simulink model "workingGT3nomasknwithcontrol"  (R2024a)
settings: Solver=ode15s  StartTime=0.0  StopTime=3600*48  RelTol=0.0001
model workspace (MAT data in the model file):
  TempGrad = 15
  Ti = 5
  roomarea1 = 20
libraries: fl_lib x2433, nesl_utility x241, SimscapeFluids_lib x137
(part 2 of 41)

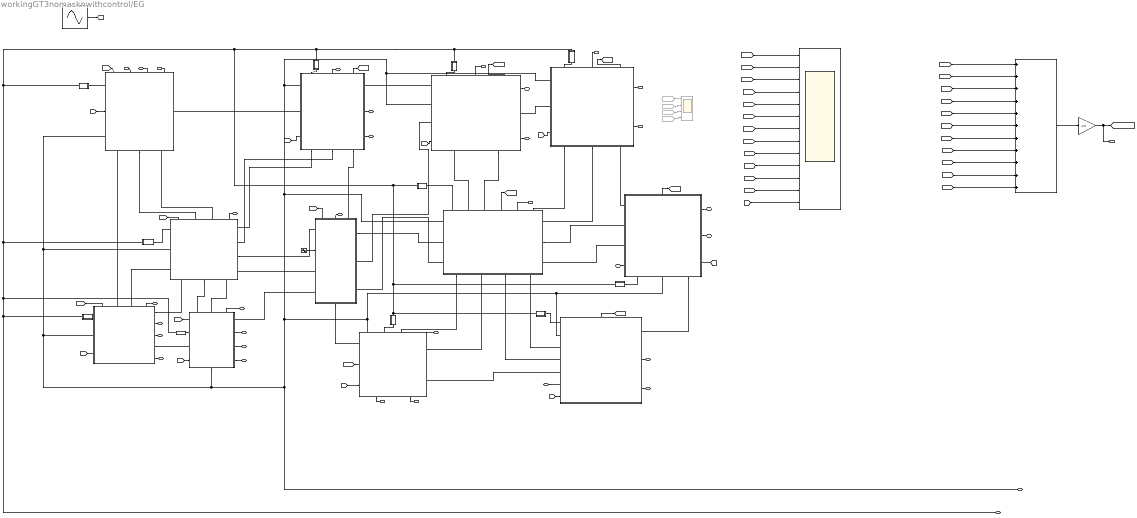
== system workingGT3nomasknwithcontrol/EG ==
  EG : Scope  NumInputPorts=13
  From : From  Commented=on  GotoTag=Troom1
  From1 : From  Commented=on  GotoTag=Troom2
  From2 : From  Commented=on  GotoTag=Troom3
  From3 : From  Commented=on  GotoTag=Troom4
  Pipe to 10 : Subsystem
  Pipe to 11 : Subsystem
  Pipe to 12 : Subsystem
  Pipe to 2 : Subsystem
  Pipe to 4 : Subsystem
  Pipe to 5 : Subsystem
  Pipe to 6 : Subsystem
  Pipe to 7 : Subsystem
  Pipe to 8 : Subsystem
  Pipe to 9a : Subsystem
  Raum1 : Subsystem
      settings: PortSchema="{\"entries\":[{\"content\":{\"sides\":[{\"content\":{\"connectorIds\":[\"LConn1\",\"LConn2\",\"LConn3\"]},\"type\":\"ConnectorPlacement.EquallySpacedRectSide\",\"uuid\":\"258852ae-79b4-4e90-ae22-4154c858ab0a\"},{\"content\":{\"connectorIds\":[\"RConn1\",\"In1\",\"RConn2\",\"RConn3\"],\"side\":\"RIGHT\"},\"type\":\"ConnectorPlacement.EquallySpacedRectSide\",\"uuid\":\"36706832-f330-42ce-9a32-f145cdee4912\"},{\"content\":{\"connectorIds\":[\"LConn4\",\"LConn5\",\"Out1\"],\"side\":\"TOP\"},\"type\":\"ConnectorPlacement.EquallySpacedRectSide\",\"uuid\":\"5cf2347a-3520-447e-9561-2d1c8313f3cf\"},{\"content\":{\"connectorIds\":[\"RConn4\"],\"side\":\"BOTTOM\"},\"type\":\"ConnectorPlacement.EquallySpacedRectSide\",\"uuid\":\"b1588268-8d41-4423-8f6e-2c28bf9b13dc\"}]},\"type\":\"ConnectorPlacement.EquallySpacedConnector\",\"uuid\":\"6bed35e7-1d7a-421b-a1f8-39267ed9017d\"}],\"packageUris\":[\"http://schema.mathworks.com/mf0/Connector/R2020b\"],\"version\":\"1.0\"}"
  Raum10 : Subsystem
      settings: PortSchema="{\"entries\":[{\"content\":{\"sides\":[{\"content\":{\"connectorIds\":[\"LConn1\",\"LConn2\",\"LConn3\",\"In1\"]},\"type\":\"ConnectorPlacement.EquallySpacedRectSide\",\"uuid\":\"258852ae-79b4-4e90-ae22-4154c858ab0a\"},{\"content\":{\"connectorIds\":[\"RConn1\",\"RConn2\",\"RConn3\"],\"side\":\"RIGHT\"},\"type\":\"ConnectorPlacement.EquallySpacedRectSide\",\"uuid\":\"36706832-f330-42ce-9a32-f145cdee4912\"},{\"content\":{\"connectorIds\":[\"LConn4\",\"LConn5\",\"Out1\"],\"side\":\"TOP\"},\"type\":\"ConnectorPlacement.EquallySpacedRectSide\",\"uuid\":\"5cf2347a-3520-447e-9561-2d1c8313f3cf\"},{\"content\":{\"connectorIds\":[\"RConn4\",\"RConn5\"],\"side\":\"BOTTOM\"},\"type\":\"ConnectorPlacement.EquallySpacedRectSide\",\"uuid\":\"b1588268-8d41-4423-8f6e-2c28bf9b13dc\"}]},\"type\":\"ConnectorPlacement.EquallySpacedConnector\",\"uuid\":\"6bed35e7-1d7a-421b-a1f8-39267ed9017d\"}],\"packageUris\":[\"http://schema.mathworks.com/mf0/Connector/R2020b\"],\"version\":\"1.0\"}"
  Raum11 : Subsystem
      settings: PortSchema="{\"entries\":[{\"content\":{\"sides\":[{\"content\":{\"connectorIds\":[\"LConn1\",\"LConn2\",\"In1\"]},\"type\":\"ConnectorPlacement.EquallySpacedRectSide\",\"uuid\":\"258852ae-79b4-4e90-ae22-4154c858ab0a\"},{\"content\":{\"connectorIds\":[\"RConn1\",\"RConn2\",\"RConn3\"],\"side\":\"RIGHT\"},\"type\":\"ConnectorPlacement.EquallySpacedRectSide\",\"uuid\":\"36706832-f330-42ce-9a32-f145cdee4912\"},{\"content\":{\"connectorIds\":[\"LConn3\",\"LConn4\",\"Out1\"],\"side\":\"TOP\"},\"type\":\"ConnectorPlacement.EquallySpacedRectSide\",\"uuid\":\"5cf2347a-3520-447e-9561-2d1c8313f3cf\"},{\"content\":{\"connectorIds\":[\"RConn4\",\"RConn5\",\"RConn6\"],\"side\":\"BOTTOM\"},\"type\":\"ConnectorPlacement.EquallySpacedRectSide\",\"uuid\":\"b1588268-8d41-4423-8f6e-2c28bf9b13dc\"}]},\"type\":\"ConnectorPlacement.EquallySpacedConnector\",\"uuid\":\"6bed35e7-1d7a-421b-a1f8-39267ed9017d\"}],\"packageUris\":[\"http://schema.mathworks.com/mf0/Connector/R2020b\"],\"version\":\"1.0\"}"
  Raum12 : Subsystem
      settings: PortSchema="{\"entries\":[{\"content\":{\"sides\":[{\"content\":{\"connectorIds\":[\"LConn1\",\"In1\",\"LConn2\"]},\"type\":\"ConnectorPlacement.EquallySpacedRectSide\",\"uuid\":\"258852ae-79b4-4e90-ae22-4154c858ab0a\"},{\"content\":{\"connectorIds\":[\"RConn1\"],\"side\":\"RIGHT\"},\"type\":\"ConnectorPlacement.EquallySpacedRectSide\",\"uuid\":\"36706832-f330-42ce-9a32-f145cdee4912\"},{\"content\":{\"connectorIds\":[\"Out1\",\"LConn3\",\"LConn4\",\"LConn5\"],\"side\":\"TOP\"},\"type\":\"ConnectorPlacement.EquallySpacedRectSide\",\"uuid\":\"5cf2347a-3520-447e-9561-2d1c8313f3cf\"},{\"content\":{\"connectorIds\":[\"RConn2\",\"RConn3\",\"RConn4\"],\"side\":\"BOTTOM\"},\"type\":\"ConnectorPlacement.EquallySpacedRectSide\",\"uuid\":\"b1588268-8d41-4423-8f6e-2c28bf9b13dc\"}]},\"type\":\"ConnectorPlacement.EquallySpacedConnector\",\"uuid\":\"6bed35e7-1d7a-421b-a1f8-39267ed9017d\"}],\"packageUris\":[\"http://schema.mathworks.com/mf0/Connector/R2020b\"],\"version\":\"1.0\"}"
  Raum2 : Subsystem
      settings: PortSchema="{\"entries\":[{\"content\":{\"sides\":[{\"content\":{\"connectorIds\":[\"LConn1\",\"LConn2\",\"LConn3\"]},\"type\":\"ConnectorPlacement.EquallySpacedRectSide\",\"uuid\":\"258852ae-79b4-4e90-ae22-4154c858ab0a\"},{\"content\":{\"connectorIds\":[\"RConn1\",\"RConn2\",\"RConn3\",\"RConn4\"],\"side\":\"RIGHT\"},\"type\":\"ConnectorPlacement.EquallySpacedRectSide\",\"uuid\":\"36706832-f330-42ce-9a32-f145cdee4912\"},{\"content\":{\"connectorIds\":[\"Out1\",\"LConn4\",\"LConn5\",\"LConn6\"],\"side\":\"TOP\"},\"type\":\"ConnectorPlacement.EquallySpacedRectSide\",\"uuid\":\"5cf2347a-3520-447e-9561-2d1c8313f3cf\"},{\"content\":{\"connectorIds\":[\"RConn5\",\"RConn6\",\"RConn7\"],\"side\":\"BOTTOM\"},\"type\":\"ConnectorPlacement.EquallySpacedRectSide\",\"uuid\":\"b1588268-8d41-4423-8f6e-2c28bf9b13dc\"}]},\"type\":\"ConnectorPlacement.EquallySpacedConnector\",\"uuid\":\"6bed35e7-1d7a-421b-a1f8-39267ed9017d\"}],\"packageUris\":[\"http://schema.mathworks.com/mf0/Connector/R2020b\"],\"version\":\"1.0\"}"
  Raum3 : Subsystem
      settings: PortSchema="{\"entries\":[{\"content\":{\"sides\":[{\"content\":{\"connectorIds\":[\"LConn1\",\"LConn2\",\"In1\"]},\"type\":\"ConnectorPlacement.EquallySpacedRectSide\",\"uuid\":\"258852ae-79b4-4e90-ae22-4154c858ab0a\"},{\"content\":{\"connectorIds\":[\"RConn1\",\"RConn2\",\"RConn3\",\"RConn4\",\"RConn5\"],\"side\":\"RIGHT\"},\"type\":\"ConnectorPlacement.EquallySpacedRectSide\",\"uuid\":\"36706832-f330-42ce-9a32-f145cdee4912\"},{\"content\":{\"connectorIds\":[\"Out1\",\"LConn3\",\"LConn4\",\"LConn5\"],\"side\":\"TOP\"},\"type\":\"ConnectorPlacement.EquallySpacedRectSide\",\"uuid\":\"5cf2347a-3520-447e-9561-2d1c8313f3cf\"},{\"content\":{\"side\":\"BOTTOM\"},\"type\":\"ConnectorPlacement.EquallySpacedRectSide\",\"uuid\":\"b1588268-8d41-4423-8f6e-2c28bf9b13dc\"}]},\"type\":\"ConnectorPlacement.EquallySpacedConnector\",\"uuid\":\"6bed35e7-1d7a-421b-a1f8-39267ed9017d\"}],\"packageUris\":[\"http://schema.mathworks.com/mf0/Connector/R2020b\"],\"version\":\"1.0\"}"
  Raum4 : Subsystem
      settings: PortSchema="{\"entries\":[{\"content\":{\"sides\":[{\"content\":{\"connectorIds\":[\"Out1\",\"LConn1\",\"LConn2\",\"In1\"]},\"type\":\"ConnectorPlacement.EquallySpacedRectSide\",\"uuid\":\"258852ae-79b4-4e90-ae22-4154c858ab0a\"},{\"content\":{\"connectorIds\":[\"RConn1\",\"RConn2\",\"RConn3\",\"RConn4\"],\"side\":\"RIGHT\"},\"type\":\"ConnectorPlacement.EquallySpacedRectSide\",\"uuid\":\"36706832-f330-42ce-9a32-f145cdee4912\"},{\"content\":{\"connectorIds\":[\"LConn3\",\"LConn4\",\"LConn5\"],\"side\":\"TOP\"},\"type\":\"ConnectorPlacement.EquallySpacedRectSide\",\"uuid\":\"5cf2347a-3520-447e-9561-2d1c8313f3cf\"},{\"content\":{\"connectorIds\":[\"RConn5\"],\"side\":\"BOTTOM\"},\"type\":\"ConnectorPlacement.EquallySpacedRectSide\",\"uuid\":\"b1588268-8d41-4423-8f6e-2c28bf9b13dc\"}]},\"type\":\"ConnectorPlacement.EquallySpacedConnector\",\"uuid\":\"6bed35e7-1d7a-421b-a1f8-39267ed9017d\"}],\"packageUris\":[\"http://schema.mathworks.com/mf0/Connector/R2020b\"],\"version\":\"1.0\"}"
  Raum5 : Subsystem
      settings: PortSchema="{\"entries\":[{\"content\":{\"sides\":[{\"content\":{\"connectorIds\":[\"LConn1\",\"LConn2\",\"LConn3\",\"LConn4\"]},\"type\":\"ConnectorPlacement.EquallySpacedRectSide\",\"uuid\":\"258852ae-79b4-4e90-ae22-4154c858ab0a\"},{\"content\":{\"connectorIds\":[\"RConn1\",\"RConn2\",\"In1\"],\"side\":\"RIGHT\"},\"type\":\"ConnectorPlacement.EquallySpacedRectSide\",\"uuid\":\"36706832-f330-42ce-9a32-f145cdee4912\"},{\"content\":{\"connectorIds\":[\"Out1\"],\"side\":\"TOP\"},\"type\":\"ConnectorPlacement.EquallySpacedRectSide\",\"uuid\":\"5cf2347a-3520-447e-9561-2d1c8313f3cf\"},{\"content\":{\"connectorIds\":[\"RConn3\",\"RConn4\",\"RConn5\"],\"side\":\"BOTTOM\"},\"type\":\"ConnectorPlacement.EquallySpacedRectSide\",\"uuid\":\"b1588268-8d41-4423-8f6e-2c28bf9b13dc\"}]},\"type\":\"ConnectorPlacement.EquallySpacedConnector\",\"uuid\":\"6bed35e7-1d7a-421b-a1f8-39267ed9017d\"}],\"packageUris\":[\"http://schema.mathworks.com/mf0/Connector/R2020b\"],\"version\":\"1.0\"}"
  Raum6 : Subsystem
      settings: PortSchema="{\"entries\":[{\"content\":{\"sides\":[{\"content\":{\"connectorIds\":[\"LConn1\",\"LConn2\",\"LConn3\",\"LConn4\",\"LConn5\",\"LConn6\",\"In1\"]},\"type\":\"ConnectorPlacement.EquallySpacedRectSide\",\"uuid\":\"258852ae-79b4-4e90-ae22-4154c858ab0a\"},{\"content\":{\"connectorIds\":[\"RConn1\",\"RConn2\",\"RConn3\"],\"side\":\"RIGHT\"},\"type\":\"ConnectorPlacement.EquallySpacedRectSide\",\"uuid\":\"36706832-f330-42ce-9a32-f145cdee4912\"},{\"content\":{\"connectorIds\":[\"Out1\"],\"side\":\"TOP\"},\"type\":\"ConnectorPlacement.EquallySpacedRectSide\",\"uuid\":\"5cf2347a-3520-447e-9561-2d1c8313f3cf\"},{\"content\":{\"side\":\"BOTTOM\"},\"type\":\"ConnectorPlacement.EquallySpacedRectSide\",\"uuid\":\"b1588268-8d41-4423-8f6e-2c28bf9b13dc\"}]},\"type\":\"ConnectorPlacement.EquallySpacedConnector\",\"uuid\":\"6bed35e7-1d7a-421b-a1f8-39267ed9017d\"}],\"packageUris\":[\"http://schema.mathworks.com/mf0/Connector/R2020b\"],\"version\":\"1.0\"}"
  Raum7 : Subsystem
      settings: PortSchema="{\"entries\":[{\"content\":{\"sides\":[{\"content\":{\"connectorIds\":[\"LConn1\",\"LConn2\",\"LConn3\"]},\"type\":\"ConnectorPlacement.EquallySpacedRectSide\",\"uuid\":\"258852ae-79b4-4e90-ae22-4154c858ab0a\"},{\"content\":{\"connectorIds\":[\"RConn1\",\"RConn2\",\"RConn3\"],\"side\":\"RIGHT\"},\"type\":\"ConnectorPlacement.EquallySpacedRectSide\",\"uuid\":\"36706832-f330-42ce-9a32-f145cdee4912\"},{\"content\":{\"connectorIds\":[\"LConn4\",\"LConn5\",\"LConn6\",\"Out1\",\"LConn7\",\"LConn8\"],\"side\":\"TOP\"},\"type\":\"ConnectorPlacement.EquallySpacedRectSide\",\"uuid\":\"5cf2347a-3520-447e-9561-2d1c8313f3cf\"},{\"content\":{\"connectorIds\":[\"RConn4\",\"RConn5\",\"RConn6\",\"RConn7\"],\"side\":\"BOTTOM\"},\"type\":\"ConnectorPlacement.EquallySpacedRectSide\",\"uuid\":\"b1588268-8d41-4423-8f6e-2c28bf9b13dc\"}]},\"type\":\"ConnectorPlacement.EquallySpacedConnector\",\"uuid\":\"6bed35e7-1d7a-421b-a1f8-39267ed9017d\"}],\"packageUris\":[\"http://schema.mathworks.com/mf0/Connector/R2020b\"],\"version\":\"1.0\"}"
  Raum8 : Subsystem
      settings: PortSchema="{\"entries\":[{\"content\":{\"sides\":[{\"content\":{\"connectorIds\":[\"LConn1\",\"Out1\",\"In1\"]},\"type\":\"ConnectorPlacement.EquallySpacedRectSide\",\"uuid\":\"258852ae-79b4-4e90-ae22-4154c858ab0a\"},{\"content\":{\"connectorIds\":[\"RConn1\",\"RConn2\"],\"side\":\"RIGHT\"},\"type\":\"ConnectorPlacement.EquallySpacedRectSide\",\"uuid\":\"36706832-f330-42ce-9a32-f145cdee4912\"},{\"content\":{\"connectorIds\":[\"LConn2\",\"LConn3\",\"LConn4\",\"LConn5\"],\"side\":\"TOP\"},\"type\":\"ConnectorPlacement.EquallySpacedRectSide\",\"uuid\":\"5cf2347a-3520-447e-9561-2d1c8313f3cf\"},{\"content\":{\"connectorIds\":[\"RConn3\",\"RConn4\"],\"side\":\"BOTTOM\"},\"type\":\"ConnectorPlacement.EquallySpacedRectSide\",\"uuid\":\"b1588268-8d41-4423-8f6e-2c28bf9b13dc\"}]},\"type\":\"ConnectorPlacement.EquallySpacedConnector\",\"uuid\":\"6bed35e7-1d7a-421b-a1f8-39267ed9017d\"}],\"packageUris\":[\"http://schema.mathworks.com/mf0/Connector/R2020b\"],\"version\":\"1.0\"}"
  Raum9 : Subsystem
      settings: PortSchema="{\"entries\":[{\"content\":{\"sides\":[{\"content\":{\"connectorIds\":[\"LConn1\",\"LConn2\",\"In1\"]},\"type\":\"ConnectorPlacement.EquallySpacedRectSide\",\"uuid\":\"258852ae-79b4-4e90-ae22-4154c858ab0a\"},{\"content\":{\"connectorIds\":[\"RConn1\",\"RConn2\"],\"side\":\"RIGHT\"},\"type\":\"ConnectorPlacement.EquallySpacedRectSide\",\"uuid\":\"36706832-f330-42ce-9a32-f145cdee4912\"},{\"content\":{\"connectorIds\":[\"LConn3\",\"LConn4\",\"Out1\"],\"side\":\"TOP\"},\"type\":\"ConnectorPlacement.EquallySpacedRectSide\",\"uuid\":\"5cf2347a-3520-447e-9561-2d1c8313f3cf\"},{\"content\":{\"connectorIds\":[\"RConn3\",\"RConn4\",\"RConn5\"],\"side\":\"BOTTOM\"},\"type\":\"ConnectorPlacement.EquallySpacedRectSide\",\"uuid\":\"b1588268-8d41-4423-8f6e-2c28bf9b13dc\"}]},\"type\":\"ConnectorPlacement.EquallySpacedConnector\",\"uuid\":\"6bed35e7-1d7a-421b-a1f8-39267ed9017d\"}],\"packageUris\":[\"http://schema.mathworks.com/mf0/Connector/R2020b\"],\"version\":\"1.0\"}"
  RaumTemperaturverlauf : Scope  Commented=on  NumInputPorts=4
  Sum of Elements : Sum  Inputs=+++++++++++
  Tatm11 : Sin  Amplitude=12  Frequency=2*pi/(24*3600)  Phase=-0.5*pi  SampleTime=0
  Tatm12 : Sin  Amplitude=7  Bias=5  Frequency=2*pi/(24*3600)  SampleTime=0
  TavgEG : Gain  Gain=1/11
  pipe to 3 : Subsystem
  hot water in : PMIOPort  Side=Left
  Y-1 : PMIOPort  Port=2  Side=Right
  Y-3 : PMIOPort  Port=3  Side=Right
  Y-4 : PMIOPort  Port=4  Side=Right
  Y-5 : PMIOPort  Port=5  Side=Right
  Y-6 : PMIOPort  Port=6  Side=Right
  Y-8 : PMIOPort  Port=7  Side=Right
  Y-7 : PMIOPort  Port=8  Side=Right
  Y-9 : PMIOPort  Port=9  Side=Right
  Y-10 : PMIOPort  Port=10  Side=Right
  Y-11 : PMIOPort  Port=11  Side=Right
  Y-12 : PMIOPort  Port=12  Side=Right
  Y-13 : PMIOPort  Port=13  Side=Right
  Y-14 : PMIOPort  Port=14  Side=Right
  Y-15 : PMIOPort  Port=15  Side=Right
  Y-16 : PMIOPort  Port=16  Side=Right
  Y-17 : PMIOPort  Port=17  Side=Right
  Y-18 : PMIOPort  Port=18  Side=Right
  Y-19 : PMIOPort  Port=19  Side=Right
  Y-20 : PMIOPort  Port=20  Side=Right
  Y-21 : PMIOPort  Port=21  Side=Right
  Hot Water Out1 : PMIOPort  Port=22  Side=Right
  Y-6 Flur12OG2 : PMIOPort  Port=23  Side=Right
  Y-Flur11OG2 : PMIOPort  Port=24  Side=Right
  Y-Flur10OG2 : PMIOPort  Port=25  Side=Right
  Y-Flur9OG2 : PMIOPort  Port=26  Side=Right
  Y-Flur8OG2 : PMIOPort  Port=27  Side=Right
  Y-Flur7OG2 : PMIOPort  Port=28  Side=Right
  Y-Flur6OG2 : PMIOPort  Port=29  Side=Right
  Y-Flur5OG2 : PMIOPort  Port=30  Side=Right
  Y-Flur4OG2 : PMIOPort  Port=31  Side=Right
  Y-Flur3OG2 : PMIOPort  Port=32  Side=Right
  Y-Flur2OG2 : PMIOPort  Port=33  Side=Right
  Y-Flur1OG2 : PMIOPort  Port=34  Side=Right
  Output : Outport
  wires:
  Raum9/1(Troom) -> [Traum9]
  [Traum4] -> EG/4
  [Traum10] -> EG/10
  [Tatm] -> Raum11/1(Tatm)
  Raum6/1(Troom) -> [Traum6]
  [Traum5] -> EG/5
  [Traum7] -> EG/7
  [Tatm] -> Raum9/1(Tatm)
  Raum7/1(Troom) -> [Traum7]
  [Traum9] -> EG/9
  From/1 -> RaumTemperaturverlauf/1
  [Traum12] -> EG/12
  Raum11/1(Troom) -> [Troom11]
  [Traum6] -> EG/6
  From2/1 -> RaumTemperaturverlauf/3
  Raum2/1(Troom) -> [Traum2]
  From3/1 -> RaumTemperaturverlauf/4
  [Tatm] -> Raum10/1(Tatm)
  Tatm11/1 -> Raum1/1(Tatm)
  [Tatm] -> Raum5/1(Tatm)
  [Tatm] -> Raum3/1(Tatm)
  [Traum1] -> EG/1
  [Tatm] -> Raum4/1(Tatm)
  From1/1 -> RaumTemperaturverlauf/2
  [Traum2] -> EG/2
  Raum3/1(Troom) -> [Traum3]
  Raum10/1(Troom) -> [Traum10]
  Raum1/1(Troom) -> [Traum1]
  [Tatm] -> Raum6/1(Tatm)
  [Traum3] -> EG/3
  [Tatm] -> Raum8/1(Tatm)
  Raum4/1(Troom) -> [Traum4]
  Raum5/1(Troom) -> [Traum5]
  [Traum8] -> EG/8
  [Troom11] -> EG/11
  Raum8/1(Troom) -> [Traum8]
  Raum12/1(Troom) -> [Traum12]
  [Tatm] -> Raum12/1(Tatm)
  Tatm12/1 -> [Tatm]
  [Troom11] -> Sum of Elements/10
  [Traum8] -> Sum of Elements/7
  [Traum3] -> Sum of Elements/2
  [Traum2] -> Sum of Elements/1
  [Traum6] -> Sum of Elements/5
  [Traum12] -> Sum of Elements/11
  [Traum9] -> Sum of Elements/8
  [Traum7] -> Sum of Elements/6
  [Traum5] -> Sum of Elements/4
  [Traum10] -> Sum of Elements/9
  [Traum4] -> Sum of Elements/3
  Sum of Elements/1 -> TavgEG/1
  TavgEG/1 -> Output/1, [TavgEG]
  [TavgEG] -> EG/13
  connections:
  Raum6/LConn5 -- Raum8/RConn2
  Raum3/LConn2 -- Raum2/LConn2 -- Raum12/LConn2 -- Raum5/RConn4 -- Raum6/LConn2 -- Raum8/LConn2 -- Raum11/LConn1 -- Raum9/LConn1 -- Raum10/LConn2 -- Raum7/LConn1 -- Hot Water Out1/RConn1 -- Raum4/RConn5
  Raum5/RConn5 -- Raum6/RConn1
  Raum7/RConn6 -- Raum6/LConn4
  Pipe to 6/RConn1 -- Raum6/LConn1
  Raum11/RConn2 -- Y-3/RConn1
  Raum1/RConn2 -- Raum2/RConn4
  Pipe to 12/RConn1 -- Raum12/LConn1
  Pipe to 7/RConn1 -- Raum7/LConn4
  Raum11/LConn2 -- Raum12/RConn1
  Pipe to 4/LConn1 -- Pipe to 2/LConn1 -- Pipe to 11/LConn1 -- Pipe to 10/LConn1 -- Pipe to 9a/LConn1 -- Pipe to 7/LConn1 -- Pipe to 6/LConn1 -- Pipe to 8/LConn1 -- Pipe to 5/LConn1 -- Pipe to 12/LConn1 -- hot water in/RConn1 -- pipe to 3/LConn1
  Raum3/LConn4 -- Raum2/LConn3
  Raum4/LConn4 -- Raum2/RConn7
  Raum10/RConn3 -- Y-9/RConn1
  Raum11/RConn6 -- Raum1/LConn4
  Raum9/LConn3 -- Pipe to 9a/RConn1
  Raum5/LConn1 -- Raum9/RConn5
  Pipe to 4/RConn1 -- Raum4/LConn1
  Raum6/RConn2 -- Y-16/RConn1
  Raum4/RConn4 -- Y-17/RConn1
  Raum3/RConn5 -- Y-18/RConn1
  Raum7/RConn7 -- Raum6/LConn3
  Pipe to 8/RConn1 -- Raum8/LConn3
  Pipe to 11/RConn1 -- Raum11/LConn3
  Raum9/RConn4 -- Raum7/RConn1
  Raum10/LConn1 -- Raum11/RConn1
  Raum8/RConn3 -- Y-20/RConn1
  Raum2/LConn5 -- Raum12/RConn4
  Raum7/LConn3 -- Raum1/LConn3
  Pipe to 10/RConn1 -- Raum10/LConn4
  Raum10/RConn1 -- Y-1/RConn1
  Raum12/LConn5 -- Y-7/RConn1
  pipe to 3/RConn1 -- Raum3/LConn1
  Raum11/RConn3 -- Y-8/RConn1
  Raum1/RConn4 -- Raum8/LConn1
  Raum9/LConn2 -- Raum10/RConn2
  Raum5/LConn3 -- Raum7/RConn3
  Raum9/RConn1 -- Y-6/RConn1
  Raum2/RConn6 -- Raum4/LConn3
  Raum7/RConn4 -- Raum8/LConn4
  Raum3/LConn3 -- Raum12/RConn2
  Raum10/LConn3 -- Raum1/LConn2
  Pipe to 2/RConn1 -- Raum2/LConn1
  Raum12/RConn3 -- Raum2/LConn4
  Raum10/RConn5 -- Raum7/LConn6
  Raum7/RConn2 -- Raum5/LConn2
  Raum11/RConn4 -- Raum2/RConn1
  Raum3/RConn1 -- Raum2/RConn5
  Raum9/RConn3 -- Raum7/LConn8
  Raum3/RConn4 -- Raum4/LConn2
  Pipe to 5/RConn1 -- Raum5/RConn3
  Raum1/RConn3 -- Raum4/RConn1
  Raum1/LConn1 -- Raum7/LConn2
  Raum11/RConn5 -- Raum2/RConn2
  Raum8/RConn1 -- Raum7/RConn5
  Raum7/LConn5 -- Raum10/RConn4
  Raum2/RConn3 -- Raum1/RConn1
  Raum4/RConn3 -- Y-15/RConn1
  Raum5/RConn1 -- Y-10/RConn1
  Raum9/RConn2 -- Y-4/RConn1
  Raum5/RConn2 -- Y-11/RConn1
  Raum8/RConn4 -- Y-21/RConn1
  Raum12/LConn3 -- Y-5/RConn1
  Raum12/LConn4 -- Y-6 Flur12OG2/RConn1
  Raum3/RConn3 -- Y-14/RConn1
  Raum3/RConn2 -- Y-12/RConn1
  Raum4/RConn2 -- Y-13/RConn1
  Raum6/RConn3 -- Y-19/RConn1
  Raum11/LConn4 -- Y-Flur11OG2/RConn1
  Raum10/LConn5 -- Y-Flur10OG2/RConn1
  Raum9/LConn4 -- Y-Flur9OG2/RConn1
  Y-Flur5OG2/RConn1 -- Raum5/LConn4
  Raum7/LConn7 -- Y-Flur7OG2/RConn1
  Y-Flur6OG2/RConn1 -- Raum6/LConn6
  Y-Flur8OG2/RConn1 -- Raum8/LConn5
  Raum1/LConn5 -- Y-Flur1OG2/RConn1
  Y-Flur4OG2/RConn1 -- Raum4/LConn5
  Raum3/LConn5 -- Y-Flur3OG2/RConn1
  Raum2/LConn6 -- Y-Flur2OG2/RConn1

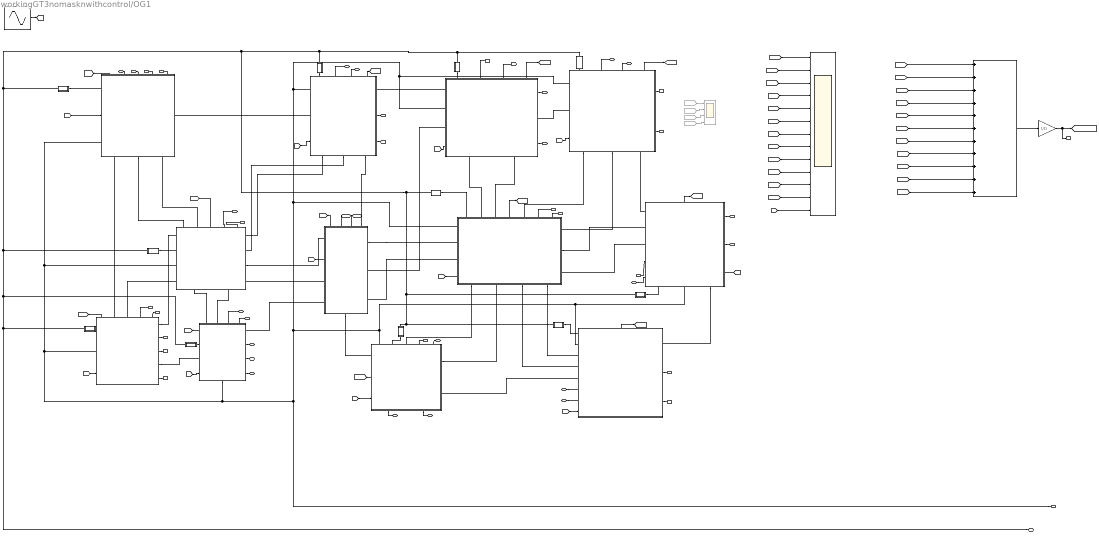
== system workingGT3nomasknwithcontrol/OG1 ==
  From : From  Commented=on  GotoTag=Troom1
  From1 : From  Commented=on  GotoTag=Troom2
  From2 : From  Commented=on  GotoTag=Troom3
  From3 : From  Commented=on  GotoTag=Troom4
  OG1 : Scope  NumInputPorts=13
  Pipe to 10 : Subsystem
  Pipe to 11 : Subsystem
  Pipe to 12 : Subsystem
  Pipe to 2 : Subsystem
  Pipe to 4 : Subsystem
  Pipe to 5 : Subsystem
  Pipe to 6 : Subsystem
  Pipe to 7 : Subsystem
  Pipe to 8 : Subsystem
  Pipe to 9a : Subsystem
  Raum1 : Subsystem
      settings: PortSchema="{\"entries\":[{\"content\":{\"sides\":[{\"content\":{\"connectorIds\":[\"LConn1\",\"LConn2\",\"LConn3\"]},\"type\":\"ConnectorPlacement.EquallySpacedRectSide\",\"uuid\":\"258852ae-79b4-4e90-ae22-4154c858ab0a\"},{\"content\":{\"connectorIds\":[\"RConn1\",\"In1\",\"RConn2\",\"RConn3\"],\"side\":\"RIGHT\"},\"type\":\"ConnectorPlacement.EquallySpacedRectSide\",\"uuid\":\"36706832-f330-42ce-9a32-f145cdee4912\"},{\"content\":{\"connectorIds\":[\"LConn4\",\"LConn5\",\"LConn6\",\"Out1\"],\"side\":\"TOP\"},\"type\":\"ConnectorPlacement.EquallySpacedRectSide\",\"uuid\":\"5cf2347a-3520-447e-9561-2d1c8313f3cf\"},{\"content\":{\"connectorIds\":[\"RConn4\"],\"side\":\"BOTTOM\"},\"type\":\"ConnectorPlacement.EquallySpacedRectSide\",\"uuid\":\"b1588268-8d41-4423-8f6e-2c28bf9b13dc\"}]},\"type\":\"ConnectorPlacement.EquallySpacedConnector\",\"uuid\":\"6bed35e7-1d7a-421b-a1f8-39267ed9017d\"}],\"packageUris\":[\"http://schema.mathworks.com/mf0/Connector/R2020b\"],\"version\":\"1.0\"}"
  Raum10 : Subsystem
      settings: PortSchema="{\"entries\":[{\"content\":{\"sides\":[{\"content\":{\"connectorIds\":[\"LConn1\",\"LConn2\",\"LConn3\",\"In1\"]},\"type\":\"ConnectorPlacement.EquallySpacedRectSide\",\"uuid\":\"258852ae-79b4-4e90-ae22-4154c858ab0a\"},{\"content\":{\"connectorIds\":[\"RConn1\",\"RConn2\",\"RConn3\"],\"side\":\"RIGHT\"},\"type\":\"ConnectorPlacement.EquallySpacedRectSide\",\"uuid\":\"36706832-f330-42ce-9a32-f145cdee4912\"},{\"content\":{\"connectorIds\":[\"LConn4\",\"LConn5\",\"LConn6\",\"Out1\"],\"side\":\"TOP\"},\"type\":\"ConnectorPlacement.EquallySpacedRectSide\",\"uuid\":\"5cf2347a-3520-447e-9561-2d1c8313f3cf\"},{\"content\":{\"connectorIds\":[\"RConn4\",\"RConn5\"],\"side\":\"BOTTOM\"},\"type\":\"ConnectorPlacement.EquallySpacedRectSide\",\"uuid\":\"b1588268-8d41-4423-8f6e-2c28bf9b13dc\"}]},\"type\":\"ConnectorPlacement.EquallySpacedConnector\",\"uuid\":\"6bed35e7-1d7a-421b-a1f8-39267ed9017d\"}],\"packageUris\":[\"http://schema.mathworks.com/mf0/Connector/R2020b\"],\"version\":\"1.0\"}"
  Raum11 : Subsystem
      settings: PortSchema="{\"entries\":[{\"content\":{\"sides\":[{\"content\":{\"connectorIds\":[\"LConn1\",\"LConn2\",\"In1\"]},\"type\":\"ConnectorPlacement.EquallySpacedRectSide\",\"uuid\":\"258852ae-79b4-4e90-ae22-4154c858ab0a\"},{\"content\":{\"connectorIds\":[\"RConn1\",\"RConn2\",\"RConn3\"],\"side\":\"RIGHT\"},\"type\":\"ConnectorPlacement.EquallySpacedRectSide\",\"uuid\":\"36706832-f330-42ce-9a32-f145cdee4912\"},{\"content\":{\"connectorIds\":[\"LConn3\",\"LConn4\",\"LConn5\",\"Out1\"],\"side\":\"TOP\"},\"type\":\"ConnectorPlacement.EquallySpacedRectSide\",\"uuid\":\"5cf2347a-3520-447e-9561-2d1c8313f3cf\"},{\"content\":{\"connectorIds\":[\"RConn4\",\"RConn5\",\"RConn6\"],\"side\":\"BOTTOM\"},\"type\":\"ConnectorPlacement.EquallySpacedRectSide\",\"uuid\":\"b1588268-8d41-4423-8f6e-2c28bf9b13dc\"}]},\"type\":\"ConnectorPlacement.EquallySpacedConnector\",\"uuid\":\"6bed35e7-1d7a-421b-a1f8-39267ed9017d\"}],\"packageUris\":[\"http://schema.mathworks.com/mf0/Connector/R2020b\"],\"version\":\"1.0\"}"
  Raum12 : Subsystem
      settings: PortSchema="{\"entries\":[{\"content\":{\"sides\":[{\"content\":{\"connectorIds\":[\"LConn1\",\"In1\",\"LConn2\"]},\"type\":\"ConnectorPlacement.EquallySpacedRectSide\",\"uuid\":\"258852ae-79b4-4e90-ae22-4154c858ab0a\"},{\"content\":{\"connectorIds\":[\"RConn1\"],\"side\":\"RIGHT\"},\"type\":\"ConnectorPlacement.EquallySpacedRectSide\",\"uuid\":\"36706832-f330-42ce-9a32-f145cdee4912\"},{\"content\":{\"connectorIds\":[\"Out1\",\"LConn3\",\"LConn4\",\"LConn5\",\"LConn6\"],\"side\":\"TOP\"},\"type\":\"ConnectorPlacement.EquallySpacedRectSide\",\"uuid\":\"5cf2347a-3520-447e-9561-2d1c8313f3cf\"},{\"content\":{\"connectorIds\":[\"RConn2\",\"RConn3\",\"RConn4\"],\"side\":\"BOTTOM\"},\"type\":\"ConnectorPlacement.EquallySpacedRectSide\",\"uuid\":\"b1588268-8d41-4423-8f6e-2c28bf9b13dc\"}]},\"type\":\"ConnectorPlacement.EquallySpacedConnector\",\"uuid\":\"6bed35e7-1d7a-421b-a1f8-39267ed9017d\"}],\"packageUris\":[\"http://schema.mathworks.com/mf0/Connector/R2020b\"],\"version\":\"1.0\"}"
  Raum2 : Subsystem
      settings: PortSchema="{\"entries\":[{\"content\":{\"sides\":[{\"content\":{\"connectorIds\":[\"LConn1\",\"LConn2\",\"LConn3\",\"LConn4\"]},\"type\":\"ConnectorPlacement.EquallySpacedRectSide\",\"uuid\":\"258852ae-79b4-4e90-ae22-4154c858ab0a\"},{\"content\":{\"connectorIds\":[\"RConn1\",\"RConn2\",\"RConn3\",\"RConn4\"],\"side\":\"RIGHT\"},\"type\":\"ConnectorPlacement.EquallySpacedRectSide\",\"uuid\":\"36706832-f330-42ce-9a32-f145cdee4912\"},{\"content\":{\"connectorIds\":[\"LConn5\",\"LConn6\",\"Out1\",\"LConn7\",\"LConn8\"],\"side\":\"TOP\"},\"type\":\"ConnectorPlacement.EquallySpacedRectSide\",\"uuid\":\"5cf2347a-3520-447e-9561-2d1c8313f3cf\"},{\"content\":{\"connectorIds\":[\"RConn5\",\"RConn6\"],\"side\":\"BOTTOM\"},\"type\":\"ConnectorPlacement.EquallySpacedRectSide\",\"uuid\":\"b1588268-8d41-4423-8f6e-2c28bf9b13dc\"}]},\"type\":\"ConnectorPlacement.EquallySpacedConnector\",\"uuid\":\"6bed35e7-1d7a-421b-a1f8-39267ed9017d\"}],\"packageUris\":[\"http://schema.mathworks.com/mf0/Connector/R2020b\"],\"version\":\"1.0\"}"
  Raum3 : Subsystem
      settings: PortSchema="{\"entries\":[{\"content\":{\"sides\":[{\"content\":{\"connectorIds\":[\"LConn1\",\"LConn2\",\"In1\"]},\"type\":\"ConnectorPlacement.EquallySpacedRectSide\",\"uuid\":\"258852ae-79b4-4e90-ae22-4154c858ab0a\"},{\"content\":{\"connectorIds\":[\"RConn1\",\"RConn2\",\"RConn3\",\"RConn4\",\"RConn5\"],\"side\":\"RIGHT\"},\"type\":\"ConnectorPlacement.EquallySpacedRectSide\",\"uuid\":\"36706832-f330-42ce-9a32-f145cdee4912\"},{\"content\":{\"connectorIds\":[\"Out1\",\"LConn3\",\"LConn4\",\"LConn5\",\"LConn6\"],\"side\":\"TOP\"},\"type\":\"ConnectorPlacement.EquallySpacedRectSide\",\"uuid\":\"5cf2347a-3520-447e-9561-2d1c8313f3cf\"},{\"content\":{\"side\":\"BOTTOM\"},\"type\":\"ConnectorPlacement.EquallySpacedRectSide\",\"uuid\":\"b1588268-8d41-4423-8f6e-2c28bf9b13dc\"}]},\"type\":\"ConnectorPlacement.EquallySpacedConnector\",\"uuid\":\"6bed35e7-1d7a-421b-a1f8-39267ed9017d\"}],\"packageUris\":[\"http://schema.mathworks.com/mf0/Connector/R2020b\"],\"version\":\"1.0\"}"
  Raum4 : Subsystem
      settings: PortSchema="{\"entries\":[{\"content\":{\"sides\":[{\"content\":{\"connectorIds\":[\"Out1\",\"LConn1\",\"LConn2\",\"In1\"]},\"type\":\"ConnectorPlacement.EquallySpacedRectSide\",\"uuid\":\"258852ae-79b4-4e90-ae22-4154c858ab0a\"},{\"content\":{\"connectorIds\":[\"RConn1\",\"RConn2\",\"RConn3\",\"RConn4\"],\"side\":\"RIGHT\"},\"type\":\"ConnectorPlacement.EquallySpacedRectSide\",\"uuid\":\"36706832-f330-42ce-9a32-f145cdee4912\"},{\"content\":{\"connectorIds\":[\"LConn3\",\"LConn4\",\"LConn5\",\"LConn6\"],\"side\":\"TOP\"},\"type\":\"ConnectorPlacement.EquallySpacedRectSide\",\"uuid\":\"5cf2347a-3520-447e-9561-2d1c8313f3cf\"},{\"content\":{\"connectorIds\":[\"RConn5\"],\"side\":\"BOTTOM\"},\"type\":\"ConnectorPlacement.EquallySpacedRectSide\",\"uuid\":\"b1588268-8d41-4423-8f6e-2c28bf9b13dc\"}]},\"type\":\"ConnectorPlacement.EquallySpacedConnector\",\"uuid\":\"6bed35e7-1d7a-421b-a1f8-39267ed9017d\"}],\"packageUris\":[\"http://schema.mathworks.com/mf0/Connector/R2020b\"],\"version\":\"1.0\"}"
  Raum5 : Subsystem
      settings: PortSchema="{\"entries\":[{\"content\":{\"sides\":[{\"content\":{\"connectorIds\":[\"LConn1\",\"LConn2\",\"LConn3\",\"LConn4\",\"LConn5\"]},\"type\":\"ConnectorPlacement.EquallySpacedRectSide\",\"uuid\":\"258852ae-79b4-4e90-ae22-4154c858ab0a\"},{\"content\":{\"connectorIds\":[\"RConn1\",\"RConn2\",\"In1\"],\"side\":\"RIGHT\"},\"type\":\"ConnectorPlacement.EquallySpacedRectSide\",\"uuid\":\"36706832-f330-42ce-9a32-f145cdee4912\"},{\"content\":{\"connectorIds\":[\"Out1\"],\"side\":\"TOP\"},\"type\":\"ConnectorPlacement.EquallySpacedRectSide\",\"uuid\":\"5cf2347a-3520-447e-9561-2d1c8313f3cf\"},{\"content\":{\"connectorIds\":[\"RConn3\",\"RConn4\",\"RConn5\"],\"side\":\"BOTTOM\"},\"type\":\"ConnectorPlacement.EquallySpacedRectSide\",\"uuid\":\"b1588268-8d41-4423-8f6e-2c28bf9b13dc\"}]},\"type\":\"ConnectorPlacement.EquallySpacedConnector\",\"uuid\":\"6bed35e7-1d7a-421b-a1f8-39267ed9017d\"}],\"packageUris\":[\"http://schema.mathworks.com/mf0/Connector/R2020b\"],\"version\":\"1.0\"}"
  Raum6 : Subsystem
      settings: PortSchema="{\"entries\":[{\"content\":{\"sides\":[{\"content\":{\"connectorIds\":[\"LConn1\",\"LConn2\",\"LConn3\",\"LConn4\",\"LConn5\",\"LConn6\",\"LConn7\",\"In1\"]},\"type\":\"ConnectorPlacement.EquallySpacedRectSide\",\"uuid\":\"258852ae-79b4-4e90-ae22-4154c858ab0a\"},{\"content\":{\"connectorIds\":[\"RConn1\",\"RConn2\",\"RConn3\"],\"side\":\"RIGHT\"},\"type\":\"ConnectorPlacement.EquallySpacedRectSide\",\"uuid\":\"36706832-f330-42ce-9a32-f145cdee4912\"},{\"content\":{\"connectorIds\":[\"Out1\"],\"side\":\"TOP\"},\"type\":\"ConnectorPlacement.EquallySpacedRectSide\",\"uuid\":\"5cf2347a-3520-447e-9561-2d1c8313f3cf\"},{\"content\":{\"side\":\"BOTTOM\"},\"type\":\"ConnectorPlacement.EquallySpacedRectSide\",\"uuid\":\"b1588268-8d41-4423-8f6e-2c28bf9b13dc\"}]},\"type\":\"ConnectorPlacement.EquallySpacedConnector\",\"uuid\":\"6bed35e7-1d7a-421b-a1f8-39267ed9017d\"}],\"packageUris\":[\"http://schema.mathworks.com/mf0/Connector/R2020b\"],\"version\":\"1.0\"}"
  Raum7 : Subsystem
      settings: PortSchema="{\"entries\":[{\"content\":{\"sides\":[{\"content\":{\"connectorIds\":[\"LConn1\",\"LConn2\",\"LConn3\",\"In1\"]},\"type\":\"ConnectorPlacement.EquallySpacedRectSide\",\"uuid\":\"258852ae-79b4-4e90-ae22-4154c858ab0a\"},{\"content\":{\"connectorIds\":[\"RConn1\",\"RConn2\",\"RConn3\"],\"side\":\"RIGHT\"},\"type\":\"ConnectorPlacement.EquallySpacedRectSide\",\"uuid\":\"36706832-f330-42ce-9a32-f145cdee4912\"},{\"content\":{\"connectorIds\":[\"LConn4\",\"LConn5\",\"LConn6\",\"Out1\",\"LConn7\",\"LConn8\",\"LConn9\"],\"side\":\"TOP\"},\"type\":\"ConnectorPlacement.EquallySpacedRectSide\",\"uuid\":\"5cf2347a-3520-447e-9561-2d1c8313f3cf\"},{\"content\":{\"connectorIds\":[\"RConn4\",\"RConn5\",\"RConn6\",\"RConn7\"],\"side\":\"BOTTOM\"},\"type\":\"ConnectorPlacement.EquallySpacedRectSide\",\"uuid\":\"b1588268-8d41-4423-8f6e-2c28bf9b13dc\"}]},\"type\":\"ConnectorPlacement.EquallySpacedConnector\",\"uuid\":\"6bed35e7-1d7a-421b-a1f8-39267ed9017d\"}],\"packageUris\":[\"http://schema.mathworks.com/mf0/Connector/R2020b\"],\"version\":\"1.0\"}"
  Raum8 : Subsystem
      settings: PortSchema="{\"entries\":[{\"content\":{\"sides\":[{\"content\":{\"connectorIds\":[\"LConn1\",\"Out1\",\"In1\"]},\"type\":\"ConnectorPlacement.EquallySpacedRectSide\",\"uuid\":\"258852ae-79b4-4e90-ae22-4154c858ab0a\"},{\"content\":{\"connectorIds\":[\"RConn1\",\"RConn2\"],\"side\":\"RIGHT\"},\"type\":\"ConnectorPlacement.EquallySpacedRectSide\",\"uuid\":\"36706832-f330-42ce-9a32-f145cdee4912\"},{\"content\":{\"connectorIds\":[\"LConn2\",\"LConn3\",\"LConn4\",\"LConn5\",\"LConn6\"],\"side\":\"TOP\"},\"type\":\"ConnectorPlacement.EquallySpacedRectSide\",\"uuid\":\"5cf2347a-3520-447e-9561-2d1c8313f3cf\"},{\"content\":{\"connectorIds\":[\"RConn3\",\"RConn4\"],\"side\":\"BOTTOM\"},\"type\":\"ConnectorPlacement.EquallySpacedRectSide\",\"uuid\":\"b1588268-8d41-4423-8f6e-2c28bf9b13dc\"}]},\"type\":\"ConnectorPlacement.EquallySpacedConnector\",\"uuid\":\"6bed35e7-1d7a-421b-a1f8-39267ed9017d\"}],\"packageUris\":[\"http://schema.mathworks.com/mf0/Connector/R2020b\"],\"version\":\"1.0\"}"
  Raum9 : Subsystem
      settings: PortSchema="{\"entries\":[{\"content\":{\"sides\":[{\"content\":{\"connectorIds\":[\"LConn1\",\"LConn2\",\"In1\"]},\"type\":\"ConnectorPlacement.EquallySpacedRectSide\",\"uuid\":\"258852ae-79b4-4e90-ae22-4154c858ab0a\"},{\"content\":{\"connectorIds\":[\"RConn1\",\"RConn2\"],\"side\":\"RIGHT\"},\"type\":\"ConnectorPlacement.EquallySpacedRectSide\",\"uuid\":\"36706832-f330-42ce-9a32-f145cdee4912\"},{\"content\":{\"connectorIds\":[\"LConn3\",\"LConn4\",\"LConn5\",\"Out1\"],\"side\":\"TOP\"},\"type\":\"ConnectorPlacement.EquallySpacedRectSide\",\"uuid\":\"5cf2347a-3520-447e-9561-2d1c8313f3cf\"},{\"content\":{\"connectorIds\":[\"RConn3\",\"RConn4\",\"RConn5\"],\"side\":\"BOTTOM\"},\"type\":\"ConnectorPlacement.EquallySpacedRectSide\",\"uuid\":\"b1588268-8d41-4423-8f6e-2c28bf9b13dc\"}]},\"type\":\"ConnectorPlacement.EquallySpacedConnector\",\"uuid\":\"6bed35e7-1d7a-421b-a1f8-39267ed9017d\"}],\"packageUris\":[\"http://schema.mathworks.com/mf0/Connector/R2020b\"],\"version\":\"1.0\"}"
  RaumTemperaturverlauf : Scope  Commented=on  NumInputPorts=4
  Sum of Elements : Sum  Inputs=+++++++++++
  Tatm12 : Sin  Amplitude=7  Bias=5  Frequency=2*pi/(24*3600)  SampleTime=0
  TavgOG1 : Gain  Gain=1/11
  pipe to 3 : Subsystem
  hot water in : PMIOPort  Side=Left
  Y-Flur12EG : PMIOPort  Port=2  Side=Left
  Y-Flur11EG : PMIOPort  Port=3  Side=Left
  Y-Flur10EG : PMIOPort  Port=4  Side=Left
  Y-Flur9EGX : PMIOPort  Port=5  Side=Left
  Y-Flur8EG : PMIOPort  Port=6  Side=Left
  Y-Flur7EG : PMIOPort  Port=7  Side=Left
  Y-Flur6EGX : PMIOPort  Port=8  Side=Left
  Y-Flur5EG : PMIOPort  Port=9  Side=Left
  Y-Flur4EG : PMIOPort  Port=10  Side=Left
  Y-Flur3EG : PMIOPort  Port=11  Side=Left
  Y-Flur2EG : PMIOPort  Port=12  Side=Left
  Y-Flur1EG : PMIOPort  Port=13  Side=Left
  Y-1 : PMIOPort  Port=14  Side=Right
  Y-3 : PMIOPort  Port=15  Side=Right
  Y-4 : PMIOPort  Port=16  Side=Right
  Y-5 : PMIOPort  Port=17  Side=Right
  Y-6 : PMIOPort  Port=18  Side=Right
  Y-8 : PMIOPort  Port=19  Side=Right
  Y-7 : PMIOPort  Port=20  Side=Right
  Y-9 : PMIOPort  Port=21  Side=Right
  Y-10 : PMIOPort  Port=22  Side=Right
  Y-11 : PMIOPort  Port=23  Side=Right
  Y-12 : PMIOPort  Port=24  Side=Right
  Y-13 : PMIOPort  Port=25  Side=Right
  Y-14 : PMIOPort  Port=26  Side=Right
  Y-15 : PMIOPort  Port=27  Side=Right
  Y-16 : PMIOPort  Port=28  Side=Right
  Y-17 : PMIOPort  Port=29  Side=Right
  Y-18 : PMIOPort  Port=30  Side=Right
  Y-19 : PMIOPort  Port=31  Side=Right
  Y-20 : PMIOPort  Port=32  Side=Right
  Y-21 : PMIOPort  Port=33  Side=Right
  Hot Water Out1 : PMIOPort  Port=34  Side=Right
  Y-Flur12OG2 : PMIOPort  Port=35  Side=Right
  Y-Flur11OG2 : PMIOPort  Port=36  Side=Right
  Y-Flur10OG2 : PMIOPort  Port=37  Side=Right
  Y-Flur9EG : PMIOPort  Port=38  Side=Right
  Y-Flur8OG2 : PMIOPort  Port=39  Side=Right
  Y-Flur7OG2 : PMIOPort  Port=40  Side=Right
  Y-Flur6EG : PMIOPort  Port=41  Side=Right
  Y-Flur5OG2 : PMIOPort  Port=42  Side=Right
  Y-Flur4OG2 : PMIOPort  Port=43  Side=Right
  Y-Flur3OG2 : PMIOPort  Port=44  Side=Right
  Y-Flur2OG2 : PMIOPort  Port=45  Side=Right
  Y-Flur1OG2 : PMIOPort  Port=46  Side=Right
  Outport : Outport
  wires:
  [Tatm] -> Raum12/1(Tatm)
  Raum12/1(Troom) -> [Traum12]
  Raum8/1(Troom) -> [Traum8]
  [Troom11] -> OG1/11
  [Traum8] -> OG1/8
  Raum5/1(Troom) -> [Traum5]
  Raum4/1(Troom) -> [Traum4]
  [Tatm] -> Raum8/1(Tatm)
  [Traum3] -> OG1/3
  [Tatm] -> Raum6/1(Tatm)
  Raum1/1(Troom) -> [Traum1]
  Raum10/1(Troom) -> [Traum10]
  Raum3/1(Troom) -> [Traum3]
  [Traum2] -> OG1/2
  From1/1 -> RaumTemperaturverlauf/2
  [Tatm] -> Raum4/1(Tatm)
  [Traum1] -> OG1/1
  [Tatm] -> Raum3/1(Tatm)
  [Tatm] -> Raum5/1(Tatm)
  [Tatm] -> Raum1/1(Tatm)
  [Tatm] -> Raum10/1(Tatm)
  From3/1 -> RaumTemperaturverlauf/4
  Raum2/1(Troom) -> [Traum2]
  From2/1 -> RaumTemperaturverlauf/3
  [Traum6] -> OG1/6
  Raum11/1(Troom) -> [Troom11]
  [Traum12] -> OG1/12
  From/1 -> RaumTemperaturverlauf/1
  [Tatm] -> Raum7/1(Tatm)
  [Traum9] -> OG1/9
  Raum7/1(Troom) -> [Traum7]
  [Tatm] -> Raum9/1(Tatm)
  [Traum7] -> OG1/7
  [Traum5] -> OG1/5
  Raum6/1(Troom) -> [Traum6]
  [Tatm] -> Raum11/1(Tatm)
  [Traum10] -> OG1/10
  [Traum4] -> OG1/4
  Raum9/1(Troom) -> [Traum9]
  Tatm12/1 -> [Tatm]
  [Traum3] -> Sum of Elements/2
  [Troom11] -> Sum of Elements/10
  [Traum12] -> Sum of Elements/11
  [Traum10] -> Sum of Elements/9
  [Traum7] -> Sum of Elements/6
  [Traum8] -> Sum of Elements/7
  [Traum2] -> Sum of Elements/1
  Sum of Elements/1 -> TavgOG1/1
  [Traum6] -> Sum of Elements/5
  [Traum5] -> Sum of Elements/4
  [Traum4] -> Sum of Elements/3
  TavgOG1/1 -> Outport/1, [TavgOG1]
  [Traum9] -> Sum of Elements/8
  [TavgOG1] -> OG1/13
  connections:
  Raum2/LConn7 -- Y-Flur2OG2/RConn1
  Raum3/LConn5 -- Y-Flur3OG2/RConn1
  Y-Flur4OG2/RConn1 -- Raum4/LConn5
  Raum1/LConn5 -- Y-Flur1OG2/RConn1
  Y-Flur8OG2/RConn1 -- Raum8/LConn5
  Y-Flur6EG/RConn1 -- Raum6/LConn6
  Raum7/LConn8 -- Y-Flur7OG2/RConn1
  Y-Flur5OG2/RConn1 -- Raum5/LConn4
  Raum9/LConn4 -- Y-Flur9EG/RConn1
  Raum10/LConn5 -- Y-Flur10OG2/RConn1
  Raum11/LConn4 -- Y-Flur11OG2/RConn1
  Raum6/RConn3 -- Y-19/RConn1
  Raum4/RConn2 -- Y-13/RConn1
  Raum3/RConn2 -- Y-12/RConn1
  Raum3/RConn3 -- Y-14/RConn1
  Raum12/LConn4 -- Y-Flur12OG2/RConn1
  Raum12/LConn3 -- Y-5/RConn1
  Raum8/RConn4 -- Y-21/RConn1
  Raum5/RConn2 -- Y-11/RConn1
  Raum9/RConn2 -- Y-4/RConn1
  Raum5/RConn1 -- Y-10/RConn1
  Raum4/RConn3 -- Y-15/RConn1
  Raum2/RConn3 -- Raum1/RConn1
  Raum7/LConn5 -- Raum10/RConn4
  Raum8/RConn1 -- Raum7/RConn5
  Raum11/RConn5 -- Raum2/RConn2
  Raum1/LConn1 -- Raum7/LConn2
  Raum1/RConn3 -- Raum4/RConn1
  Pipe to 5/RConn1 -- Raum5/RConn3
  Raum3/RConn4 -- Raum4/LConn2
  Raum9/RConn3 -- Raum7/LConn7
  Raum3/RConn1 -- Raum2/LConn1
  Raum11/RConn4 -- Raum2/RConn1
  Raum7/RConn2 -- Raum5/LConn2
  Raum10/RConn5 -- Raum7/LConn6
  Raum12/RConn3 -- Raum2/LConn5
  Pipe to 2/RConn1 -- Raum2/LConn2
  Raum10/LConn3 -- Raum1/LConn2
  Raum3/LConn3 -- Raum12/RConn2
  Raum7/RConn4 -- Raum8/LConn4
  Raum2/RConn5 -- Raum4/LConn3
  Raum9/RConn1 -- Y-6/RConn1
  Raum5/LConn3 -- Raum7/RConn3
  Raum9/LConn2 -- Raum10/RConn2
  Raum1/RConn4 -- Raum8/LConn1
  Raum11/RConn3 -- Y-8/RConn1
  pipe to 3/RConn1 -- Raum3/LConn1
  Raum12/LConn6 -- Y-7/RConn1
  Raum10/RConn1 -- Y-1/RConn1
  Pipe to 10/RConn1 -- Raum10/LConn4
  Raum7/LConn3 -- Raum1/LConn3
  Raum2/LConn6 -- Raum12/RConn4
  Raum8/RConn3 -- Y-20/RConn1
  Raum10/LConn1 -- Raum11/RConn1
  Raum9/RConn4 -- Raum7/RConn1
  Pipe to 11/RConn1 -- Raum11/LConn3
  Pipe to 8/RConn1 -- Raum8/LConn3
  Raum7/RConn7 -- Raum6/LConn3
  Raum3/RConn5 -- Y-18/RConn1
  Raum4/RConn4 -- Y-17/RConn1
  Raum6/RConn2 -- Y-16/RConn1
  Pipe to 4/RConn1 -- Raum4/LConn1
  Raum5/LConn1 -- Raum9/RConn5
  Raum9/LConn3 -- Pipe to 9a/RConn1
  Raum11/RConn6 -- Raum1/LConn4
  Raum10/RConn3 -- Y-9/RConn1
  Raum4/LConn4 -- Raum2/RConn6
  Raum3/LConn4 -- Raum2/LConn4
  hot water in/RConn1 -- pipe to 3/LConn1 -- Pipe to 12/LConn1 -- Pipe to 5/LConn1 -- Pipe to 8/LConn1 -- Pipe to 6/LConn1 -- Pipe to 7/LConn1 -- Pipe to 9a/LConn1 -- Pipe to 10/LConn1 -- Pipe to 11/LConn1 -- Pipe to 2/LConn1 -- Pipe to 4/LConn1
  Raum11/LConn2 -- Raum12/RConn1
  Pipe to 7/RConn1 -- Raum7/LConn4
  Pipe to 12/RConn1 -- Raum12/LConn1
  Raum1/RConn2 -- Raum2/RConn4
  Raum11/RConn2 -- Y-3/RConn1
  Pipe to 6/RConn1 -- Raum6/LConn1
  Raum7/RConn6 -- Raum6/LConn4
  Raum5/RConn5 -- Raum6/RConn1
  Hot Water Out1/RConn1 -- Raum7/LConn1 -- Raum10/LConn2 -- Raum9/LConn1 -- Raum11/LConn1 -- Raum8/LConn2 -- Raum6/LConn2 -- Raum5/RConn4 -- Raum4/RConn5 -- Raum12/LConn2 -- Raum2/LConn3 -- Raum3/LConn2
  Raum6/LConn5 -- Raum8/RConn2
  Raum1/LConn6 -- Y-Flur1EG/RConn1
  Raum3/LConn6 -- Y-Flur3EG/RConn1
  Raum4/LConn6 -- Y-Flur4EG/RConn1
  Y-Flur5EG/RConn1 -- Raum5/LConn5
  Y-Flur6EGX/RConn1 -- Raum6/LConn7
  Raum7/LConn9 -- Y-Flur7EG/RConn1
  Raum8/LConn6 -- Y-Flur8EG/RConn1
  Raum9/LConn5 -- Y-Flur9EGX/RConn1
  Raum10/LConn6 -- Y-Flur10EG/RConn1
  Raum11/LConn5 -- Y-Flur11EG/RConn1
  Raum12/LConn5 -- Y-Flur12EG/RConn1
  Raum2/LConn8 -- Y-Flur2EG/RConn1
